simulink model "SmartGridSimulation"  (R2023a)
settings: Solver=VariableStepAuto  StartTime=0.0  StopTime=10  RelTol=1e-3
undefined symbols (not defined in the file or in its folder): Ion, Lithium
libraries: spsSeriesRLCBranchLib x7, spsCurrentMeasurementLib x2, spsMosfetLib x2, spsPWMGeneratorDCDCLib x2, spsVoltageMeasurementLib x2, spsBatteryLib x1, slpidlib x1, simulink x1, spsPVArrayLib x1, spsDiodeLib x1, spsIGBTDiodeLib x1, spspowerguiLib x1
settings Model: Creator=DISHAN  LastModifiedBy=Dishan Dey
settings SolverCC: ZeroCrossAlgorithm=Adaptive
settings DebuggingCC: MaskedZcDiagnostic=none  IgnoredZcDiagnostic=none

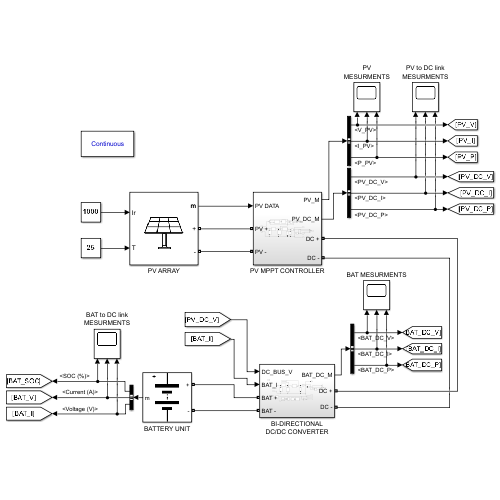
[thumbnail: Simulink's stored preview of the top-level diagram]
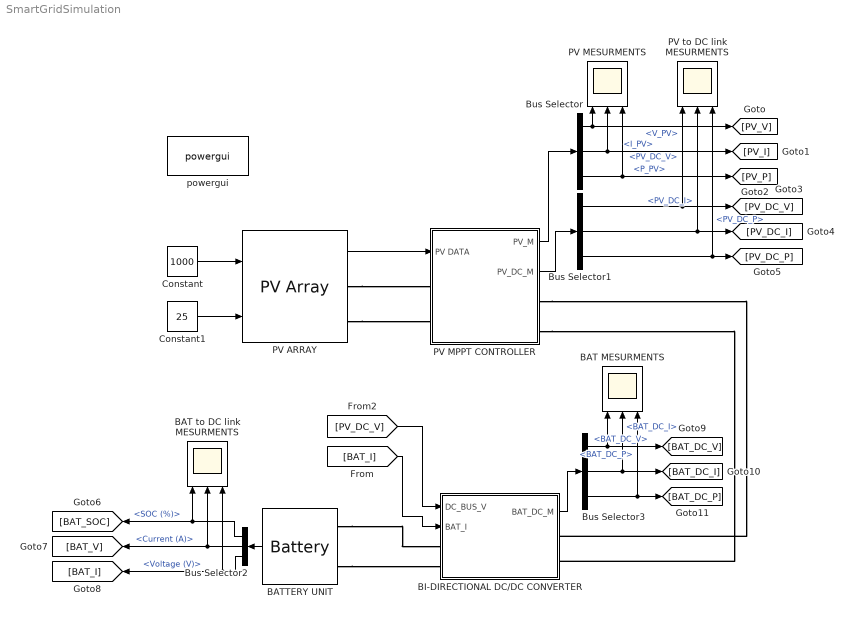
== system SmartGridSimulation ==
  BAT MESURMENTS : Scope  NumInputPorts=3
  BAT to DC link MESURMENTS : Scope  NumInputPorts=3
  BATTERY UNIT : spsBatteryLib/Battery  BatType=Lithium-Ion  ShowTempParam=off  ThermalPreset=no  ShowAgeParam=off  NomV=12*35  NomQ=5000  SOC=50  Batt_Tr=0.0001  PresetModel=on  MaxQ=5000  MinV=315  FullV=488.8746  Dis_rate=2173.913  R=0.00084  Normal_OP=4521.7391  expZone="[453.7621      245.6522]"  current=[6.5 13 32.5]  Units=Time  Tci=20  NomT=20  T2=-30  MaxQ2=4.8  FullV2=7.1  Normal_OP2=5.655  expZone2="[6.58           1]"  Rca=0.6  ti=2000  Dp=0  Neq0=0  Tsim=1e6  Ta1=25  Qeol=5.4*0.9  Reol=0.013333*1.2  Char_age=[2.3478, 3]  Dis_age=[2.3478, 10]  N1=1500  N2=10500  N3=1000  N4=1400  Ta2=45  N5=950
  BI-DIRECTIONAL DC/DC CONVERTER : Subsystem
  Bus Selector : BusSelector  OutputSignals=V_PV,I_PV,P_PV
  Bus Selector1 : BusSelector  OutputSignals=PV_DC_V,PV_DC_I,PV_DC_P
  Bus Selector2 : BusSelector  OutputSignals=SOC (%),Current (A),Voltage (V)
  Bus Selector3 : BusSelector  OutputSignals=BAT_DC_V,BAT_DC_I,BAT_DC_P
  Constant : Constant  Value=1000
  Constant1 : Constant  Value=25
  PV MESURMENTS : Scope  NumInputPorts=3
  PV ARRAY : spsPVArrayLib/PV Array  Npar=1300  Nser=11  PlotType=array @ 25 deg.C & specified irradiances  S_vec="[ 1000  500  100 ]"  Temp_C_vec="[ 45 25  ]"  ModuleName=User-defined  PlotWhenSelected=off  Pm=213.15  Ncell=60  Voc=36.3  Isc=7.84  Vm=29  Im=7.35  beta_Voc_pc=-0.36099  alpha_Isc_pc=0.102  beta_Voc=-0.13104  alpha_Isc=0.0079968  IL=7.8654  I0=2.9273e-10  nI=0.98119  Rsh=313.0553  Rs=0.39381  RobustModel=off  RobustCellTemperature=313.3991  BAL=on  Tc=1e-6  Tfilter=5e-5
  PV MPPT CONTROLLER : Subsystem
  PV to DC link MESURMENTS : Scope  NumInputPorts=3
  powergui : spspowerguiLib/powergui  Priority=1  SimulationMode=Continuous  SampleTime=5e-05  frequency=60  Iterations=50  frequencyindice=0  Pbase=100e6  ErrMax=1e-4  UnitsV=kV  UnitsW=MW  buscounter=0  FunctionMessages=off  echomessages=off  EnableUseOfTLC=off  CurrentSourceSwitches=off  DisableSnubberDevices=off  DisableRonSwitches=off  DisableVfSwitches=off  DisplayEquations=off  AutomaticDiscreteSolvers=off  SolverType=Tustin/Backward Euler (TBE)  Interpol=off  ExternalGateDelay=off  methode=off  Ts=100  x0status=blocks  SPID=on  SwTol=0  HookPort=off  NonlinearTolerance=1e-4  nMaxIteration=100  ContinueOnMaxIteration=off  RestoreLinks=warning  ResistiveCurrentMeasurement=off  Frange=[0:2:500]  Ylog=off  Xlog=on  ShowGrid=off  save=off  variable=ZData  structure=0  ZoomFFT=off  StartTime=0.0  cycles=1  DisplayStyle=1  fundamental=60  FreqAxis=off  MaxFrequency=1000  frequencyindicesteady=1  RmsSteady=1  display=off
  wires:
  Constant/1 -> PV ARRAY/1
  Constant1/1 -> PV ARRAY/2
  PV ARRAY/1 -> PV MPPT CONTROLLER/1(PV DATA)
  PV MPPT CONTROLLER/1(PV_M) -> Bus Selector/1
  PV MPPT CONTROLLER/2(PV_DC_M) -> Bus Selector1/1
  Bus Selector/1 -> PV MESURMENTS/1, [PV_V]  "<V_PV>"
  Bus Selector/2 -> [PV_I], PV MESURMENTS/2  "<I_PV>"
  Bus Selector/3 -> [PV_P], PV MESURMENTS/3  "<P_PV>"
  Bus Selector1/1 -> [PV_DC_V], PV to DC link MESURMENTS/1  "<PV_DC_V>"
  Bus Selector1/2 -> [PV_DC_I], PV to DC link MESURMENTS/2  "<PV_DC_I>"
  Bus Selector1/3 -> [PV_DC_P], PV to DC link MESURMENTS/3  "<PV_DC_P>"
  BATTERY UNIT/1 -> Bus Selector2/1
  Bus Selector2/1 -> BAT to DC link MESURMENTS/1, [BAT_SOC]  "<SOC (%)>"
  Bus Selector2/2 -> BAT to DC link MESURMENTS/2, [BAT_V]  "<Current (A)>"
  Bus Selector2/3 -> BAT to DC link MESURMENTS/3, [BAT_I]  "<Voltage (V)>"
  Bus Selector3/2 -> BAT MESURMENTS/2, [BAT_DC_I]  "<BAT_DC_I>"
  Bus Selector3/3 -> [BAT_DC_P], BAT MESURMENTS/3  "<BAT_DC_P>"
  Bus Selector3/1 -> BAT MESURMENTS/1, [BAT_DC_V]  "<BAT_DC_V>"
  BI-DIRECTIONAL DC/DC CONVERTER/1(BAT_DC_M) -> Bus Selector3/1
  [PV_DC_V] -> BI-DIRECTIONAL DC/DC CONVERTER/1(DC_BUS_V)
  [BAT_I] -> BI-DIRECTIONAL DC/DC CONVERTER/2(BAT_I)
  connections:
  PV ARRAY/RConn1 -- PV MPPT CONTROLLER/LConn1
  PV ARRAY/RConn2 -- PV MPPT CONTROLLER/LConn2
  BATTERY UNIT/LConn1 -- BI-DIRECTIONAL DC/DC CONVERTER/LConn1
  BATTERY UNIT/LConn2 -- BI-DIRECTIONAL DC/DC CONVERTER/LConn2
  PV MPPT CONTROLLER/RConn1 -- BI-DIRECTIONAL DC/DC CONVERTER/RConn1
  PV MPPT CONTROLLER/RConn2 -- BI-DIRECTIONAL DC/DC CONVERTER/RConn2

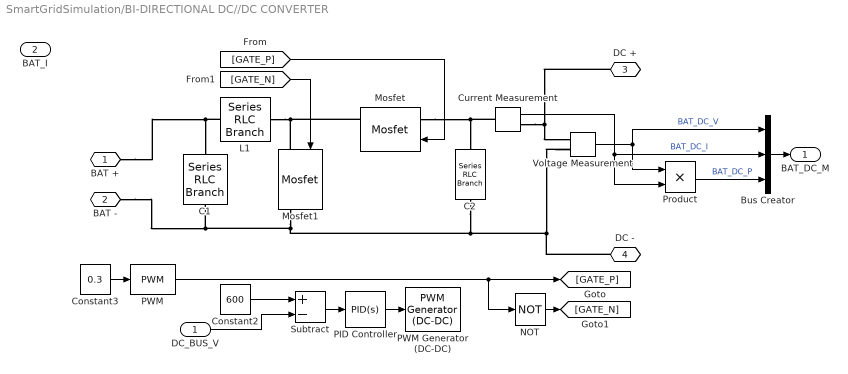
== system SmartGridSimulation/BI-DIRECTIONAL DC//DC CONVERTER ==
  DC_BUS_V : Inport
  BAT_I : Inport  Port=2
  Bus Creator : BusCreator  Inputs=3
  C1 : spsSeriesRLCBranchLib/Series RLC Branch  LConnTagsString=__new0  RConnTagsString=__new0  BranchType=RC  Resistance=1  Inductance=1e-3  SetiL0=off  InitialCurrent=0  Capacitance=64.7e-06  Setx0=off  InitialVoltage=0  Measurements=None
  C2 : spsSeriesRLCBranchLib/Series RLC Branch  LConnTagsString=__new0  RConnTagsString=__new0  BranchType=RC  Resistance=1  Inductance=1e-3  SetiL0=off  InitialCurrent=0  Capacitance=7609e-06  Setx0=off  InitialVoltage=0  Measurements=None
  Constant2 : Constant  Value=600
  Constant3 : Constant  Value=0.3
  Current Measurement : spsCurrentMeasurementLib/Current Measurement  PhasorSimulation=off  OutputType=Complex  PSBequivalent=0
  L1 : spsSeriesRLCBranchLib/Series RLC Branch  LConnTagsString=__new0  RConnTagsString=__new0  BranchType=L  Resistance=1  Inductance=579.5e-06  SetiL0=off  InitialCurrent=0  Capacitance=1e-6  Setx0=off  InitialVoltage=0  Measurements=None
  Mosfet : spsMosfetLib/Mosfet  Ron=0.1  Lon=0  Rd=0.01  Vfd=0  IC=0  Rs=1e5  Cs=inf  Measurements=on
  Mosfet1 : spsMosfetLib/Mosfet  Ron=0.1  Lon=0  Rd=0.01  Vfd=0  IC=0  Rs=1e5  Cs=inf  Measurements=on
  NOT : Logic  Operator=NOT  IconShape=distinctive  AllPortsSameDT=off  OutDataTypeStr=boolean
  PID Controller : slpidlib/PID Controller  Controller=PID  Form=Parallel  TimeDomain=Continuous-time  UseExternalTs=off  SampleTime=-1  IntegratorMethod=Forward Euler  FilterMethod=Forward Euler  ControllerParametersSource=internal  P=1  I=1  UseKiTs=off  D=0  N=100  UseFilter=on  TunerSelectOption=Transfer Function Based (PID Tuner App)  InitialConditionSource=internal  InitialConditionForIntegrator=0  InitialConditionForFilter=0  DifferentiatorICPrevScaledInput=0  ExternalReset=none  TrackingMode=off  Kt=1  LimitOutput=off  SatLimitsSource=internal  UpperSaturationLimit=inf  LowerSaturationLimit=-inf  LinearizeAsGain=on  AntiWindupMode=none  Kb=1  LimitIntegrator=off  UpperIntegratorSaturationLimit=inf  LowerIntegratorSaturationLimit=-inf  POutMin=[]  POutMax=[]  IOutMin=[]  IOutMax=[]  DOutMin=[]  DOutMax=[]  NOutMin=[]  NOutMax=[]  SumOutMin=[]  SumOutMax=[]  SaturationOutMin=[]  SaturationOutMax=[]  PParamMin=[]  PParamMax=[]  IParamMin=[]  IParamMax=[]  DParamMin=[]  DParamMax=[]  NParamMin=[]  NParamMax=[]  KbParamMin=[]  KbParamMax=[]  KtParamMin=[]  KtParamMax=[]  KbOutMin=[]  KbOutMax=[]  KtOutMin=[]  KtOutMax=[]  IntegratorOutMin=[]  IntegratorOutMax=[]  FilterOutMin=[]  FilterOutMax=[]  SumI1OutMin=[]  SumI1OutMax=[]  SumI2OutMin=[]  SumI2OutMax=[]  SumI3OutMin=[]  SumI3OutMax=[]  SumI4OutMin=[]  SumI4OutMax=[]  SumDOutMin=[]  SumDOutMax=[]  DifferentiatorOutMin=[]  DifferentiatorOutMax=[]  FilterDiffOutCoefMin=[]  FilterDiffOutCoefMax=[]  ReciprocalOutMin=[]  ReciprocalOutMax=[]  SumDenOutMin=[]  SumDenOutMax=[]  SumNumOutMin=[]  SumNumOutMax=[]  DivideOutMin=[]  DivideOutMax=[]  UdiffTsProdOutMin=[]  UdiffTsProdOutMax=[]  NTsProdOutMin=[]  NTsProdOutMax=[]  UintegralTsProdOutMin=[]  UintegralTsProdOutMax=[]  UngainTsProdOutMin=[]  UngainTsProdOutMax=[]  ClampingZeroOutDataTypeStr=Inherit: Inherit via back propagation  ClampingZeroOutMin=[]  ClampingZeroOutMax=[]  FilterDenConstantOutDataTypeStr=Inherit: Inherit via back propagation  FilterDenConstantOutMin=[]  FilterDenConstantOutMax=[]  PCopyOutDataTypeStr=Inherit: Inherit via back propagation  PCopyOutMin=[]  PCopyOutMax=[]  NCopyOutDataTypeStr=Inherit: Inherit via back propagation  NCopyOutMin=[]  NCopyOutMax=[]  IntegratorContinuousStateAttributes=''  IntegratorStateMustResolveToSignalObject=off  IntegratorRTWStateStorageClass=Auto  FilterContinuousStateAttributes=''  FilterStateMustResolveToSignalObject=off  FilterRTWStateStorageClass=Auto  ParallelPVariant=InternalParameters  IdealPVariant=Disabled  IVariant=InternalParameters  DVariant=InternalParameters  IntegratorVariant=Continuous  SatVariant=Disabled  AWVariant=Passthrough  PCopyVariant=Disabled  TRVariant=Disabled  FdbkBlocksVariant=Forward  IdealPFdbkVariant=Disabled  SatFdbkVariant=Disabled  DerivativeFilterVariant=ContFilter  NVariant=InternalParameters  NCopyVariant=Disabled  FilterICVariant=InternalICsFilter  IntegratorICVariant=InternalICs  ExternalResetVariant=Disabled  TRSumVariant=Passthrough  SumFdbkVariant=Disabled  SumVariant=Sum_PID  TsampFilterVariant=InternalTs  TsampNgainVariant=Passthrough  TsampIntegralVariant=Disabled_SignalSpec  ExternalSaturationOutDataTypeStr=Inherit: Same as second input
  PWM : simulink/Discontinuities/PWM  DisableCoverage=on  Period=1/10000  InitialDelay=0  DisallowZeroDutyCycle=off  RunAtFixedTimeIntervals=off  SampleTime=0.1
  PWM Generator (DC-DC) : spsPWMGeneratorDCDCLib/PWM Generator (DC-DC)  Fsw=10000  Ts=0
  Product : Product
  Subtract : Sum  Inputs=+-
  Voltage Measurement : spsVoltageMeasurementLib/Voltage Measurement  PhasorSimulation=off  OutputType=Complex  PSBequivalent=0
  BAT + : PMIOPort  Side=Left
  BAT - : PMIOPort  Port=2  Side=Left
  DC + : PMIOPort  Port=3  Side=Right
  DC - : PMIOPort  Port=4  Side=Right
  BAT_DC_M : Outport
  wires:
  Constant2/1 -> Subtract/1
  Product/1 -> Bus Creator/3  "BAT_DC_P"
  Bus Creator/1 -> BAT_DC_M/1
  DC_BUS_V/1 -> Subtract/2
  Subtract/1 -> PID Controller/1
  Voltage Measurement/1 -> Bus Creator/1, Product/1  "BAT_DC_V"
  Current Measurement/1 -> Product/2, Bus Creator/2  "BAT_DC_I"
  NOT/1 -> [GATE_N]
  PID Controller/1 -> PWM Generator (DC-DC)/1
  Constant3/1 -> PWM/1
  PWM/1 -> NOT/1, [GATE_P]
  [GATE_P] -> Mosfet/1
  [GATE_N] -> Mosfet1/1
  connections:
  DC -/RConn1 -- Voltage Measurement/LConn2 -- C2/RConn1 -- Mosfet1/RConn1 -- C1/RConn1 -- BAT -/RConn1
  L1/LConn1 -- Mosfet1/LConn1 -- Mosfet/RConn1
  L1/RConn1 -- C1/LConn1 -- BAT +/RConn1
  Current Measurement/LConn1 -- Mosfet/LConn1 -- C2/LConn1
  Current Measurement/RConn1 -- DC +/RConn1 -- Voltage Measurement/LConn1

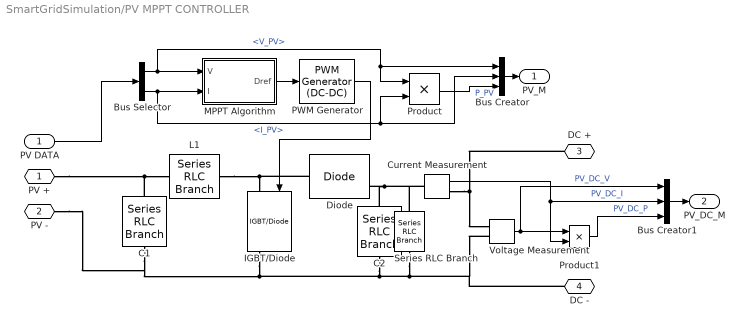
== system SmartGridSimulation/PV MPPT CONTROLLER ==
  PV DATA : Inport
  Bus Creator : BusCreator  Inputs=3
  Bus Creator1 : BusCreator  Inputs=3
  Bus Selector : BusSelector  OutputSignals=V_PV,I_PV
  C1 : spsSeriesRLCBranchLib/Series RLC Branch  LConnTagsString=__new0  RConnTagsString=__new0  BranchType=C  Resistance=1  Inductance=1e-3  SetiL0=off  InitialCurrent=0  Capacitance=0.0397  Setx0=off  InitialVoltage=0  Measurements=None
  C2 : spsSeriesRLCBranchLib/Series RLC Branch  LConnTagsString=__new0  RConnTagsString=__new0  BranchType=C  Resistance=1  Inductance=1e-3  SetiL0=off  InitialCurrent=0  Capacitance=0.0397  Setx0=off  InitialVoltage=0  Measurements=None
  Current Measurement : spsCurrentMeasurementLib/Current Measurement  PhasorSimulation=off  OutputType=Complex  PSBequivalent=0
  Diode : spsDiodeLib/Diode  Ron=0.001  Lon=0  Vf=0.8  IC=0  UseSnubber=0  Rs=500  Cs=250e-9  Measurements=on
  IGBT/Diode : spsIGBTDiodeLib/IGBT//Diode  Ron=1e-3  Rs=1e5  Cs=inf  Measurements=on
  L1 : spsSeriesRLCBranchLib/Series RLC Branch  LConnTagsString=__new0  RConnTagsString=__new0  BranchType=L  Resistance=1  Inductance=1.5636e-04  SetiL0=off  InitialCurrent=0  Capacitance=1e-6  Setx0=off  InitialVoltage=0  Measurements=None
  MPPT Algorithm : MATLAB Function  TreatAsAtomicUnit=on
  PWM Generator : spsPWMGeneratorDCDCLib/PWM Generator (DC-DC)  Fsw=10000  Ts=0
  Product : Product
  Product1 : Product
  Series RLC Branch : spsSeriesRLCBranchLib/Series RLC Branch  LConnTagsString=__new0  RConnTagsString=__new0  BranchType=R  Resistance=0.1181  Inductance=1e-3  SetiL0=off  InitialCurrent=0  Capacitance=1e-6  Setx0=off  InitialVoltage=0  Measurements=None
  Voltage Measurement : spsVoltageMeasurementLib/Voltage Measurement  PhasorSimulation=off  OutputType=Complex  PSBequivalent=0
  PV + : PMIOPort  Side=Left
  PV - : PMIOPort  Port=2  Side=Left
  DC + : PMIOPort  Port=3  Side=Right
  DC - : PMIOPort  Port=4  Side=Right
  PV_M : Outport
  PV_DC_M : Outport  Port=2
  wires:
  Bus Selector/1 -> Bus Creator/1, Product/1, MPPT Algorithm/1(V)  "<V_PV>"
  MPPT Algorithm/1(Dref) -> PWM Generator/1
  Bus Selector/2 -> Bus Creator/2, Product/2, MPPT Algorithm/2(I)  "<I_PV>"
  PV DATA/1 -> Bus Selector/1
  Product/1 -> Bus Creator/3  "P_PV"
  PWM Generator/1 -> IGBT/Diode/1
  Bus Creator/1 -> PV_M/1
  Bus Creator1/1 -> PV_DC_M/1
  Voltage Measurement/1 -> Bus Creator1/1, Product1/1  "PV_DC_V"
  Product1/1 -> Bus Creator1/3  "PV_DC_P"
  Current Measurement/1 -> Product1/2, Bus Creator1/2  "PV_DC_I"
  connections:
  PV +/RConn1 -- C1/LConn1 -- L1/RConn1
  L1/LConn1 -- Diode/LConn1 -- IGBT/Diode/LConn1
  IGBT/Diode/RConn1 -- Series RLC Branch/RConn1 -- Voltage Measurement/LConn2 -- DC -/RConn1 -- C2/RConn1 -- C1/RConn1 -- PV -/RConn1
  Diode/RConn1 -- Series RLC Branch/LConn1 -- Current Measurement/LConn1 -- C2/LConn1
  Current Measurement/RConn1 -- DC +/RConn1 -- Voltage Measurement/LConn1

== matlab function SmartGridSimulation/PV MPPT CONTROLLER/MPPT Algorithm ==
  settings: updateMethod=DISCRETE
  data: V input; Dref output; I input
function Dref = mppt(V,I)
Dini = 0.42;
Dmax = 0.9;
Dmin = 0.1;
delDref = 0.00008;

persistent Vold Pold Drefold

if(isempty(Vold))
    Vold = 0;
    Pold = 0;
    Drefold = Dini;
end

P = V*I;
delV = V - Vold;
delP = P - Pold;

    if delP>0
        if delV>0
            Dref = Drefold - delDref;
        else
            Dref = Drefold + delDref;
        end
    elseif delP<0
        if delV>0
            Dref = Drefold + delDref;
        else
            Dref = Drefold - delDref;
        end
    else
        Dref = Drefold;
    end
    
    if Dref>Dmax || Dref<Dmin
        Dref = Drefold;
    end
Drefold = Dref;
Pold = P;
Vold = V;
